simulink model "lim_s_function"  (R2017a)
settings: Solver=ode4  StartTime=0.0  StopTime=1  FixedStep=1e-5  MaxStep=1  RelTol=1e-3
settings Model: Creator=QAQ  LastModifiedBy=QAQ

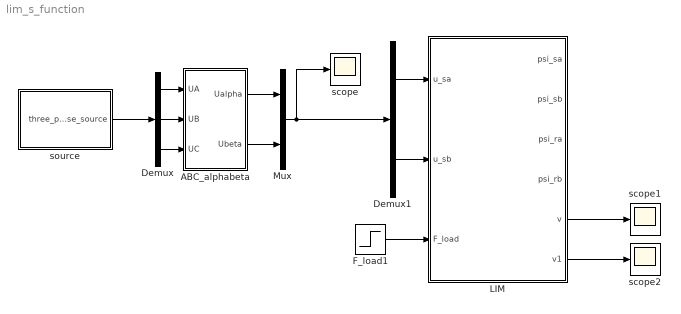
== system lim_s_function ==
  ABC_alphabeta : Subsystem
  Demux : Demux  Outputs=3
  Demux1 : Demux  Outputs=2
  F_load1 : Step  Time=0  After=1000  SampleTime=0
  LIM : Subsystem
  Mux : Mux  Inputs=2
  scope : Scope
  scope1 : Scope
  scope2 : Scope
  source : Subsystem
  wires:
  Demux/2 -> ABC_alphabeta/2(UB)
  Demux/3 -> ABC_alphabeta/3(UC)
  source/1(three_phase_source) -> Demux/1
  Mux/1 -> scope/1, Demux1/1
  ABC_alphabeta/2(Ubeta) -> Mux/2
  Demux/1 -> ABC_alphabeta/1(UA)
  Demux1/1 -> LIM/1(u_sa)
  ABC_alphabeta/1(Ualpha) -> Mux/1
  Demux1/2 -> LIM/2(u_sb)
  F_load1/1 -> LIM/3(F_load)
  LIM/5(v) -> scope1/1
  LIM/6(v1) -> scope2/1

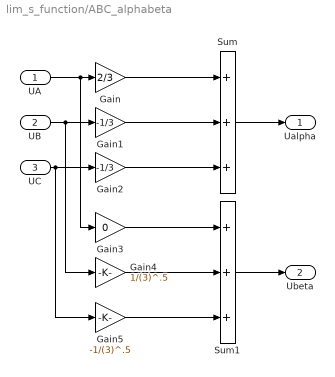
== system lim_s_function/ABC_alphabeta ==
  UA : Inport
  UB : Inport  Port=2
  UC : Inport  Port=3
  Gain : Gain  Gain=2/3  SaturateOnIntegerOverflow=on  OutDataTypeStr=Inherit: Same as input  ParamDataTypeStr=Inherit: Same as input
  Gain1 : Gain  Gain=-1/3  SaturateOnIntegerOverflow=on  OutDataTypeStr=Inherit: Same as input  ParamDataTypeStr=Inherit: Same as input
  Gain2 : Gain  Gain=-1/3  SaturateOnIntegerOverflow=on  OutDataTypeStr=Inherit: Same as input  ParamDataTypeStr=Inherit: Same as input
  Gain3 : Gain  Gain=0  SaturateOnIntegerOverflow=on  OutDataTypeStr=Inherit: Same as input  ParamDataTypeStr=Inherit: Same as input
  Gain4 : Gain  Gain=1/(3)^.5  SaturateOnIntegerOverflow=on  OutDataTypeStr=Inherit: Same as input  ParamDataTypeStr=Inherit: Same as input
  Gain5 : Gain  Gain=-1/(3)^.5  SaturateOnIntegerOverflow=on  OutDataTypeStr=Inherit: Same as input  ParamDataTypeStr=Inherit: Same as input
  Sum : Sum  Inputs=+++  SaturateOnIntegerOverflow=on
  Sum1 : Sum  Inputs=+++  SaturateOnIntegerOverflow=on
  Ualpha : Outport
  Ubeta : Outport  Port=2
  wires:
  UA/1 -> Gain3/1, Gain/1
  UB/1 -> Gain4/1, Gain1/1
  UC/1 -> Gain5/1, Gain2/1
  Gain/1 -> Sum/1
  Gain1/1 -> Sum/2
  Gain2/1 -> Sum/3
  Sum/1 -> Ualpha/1
  Gain3/1 -> Sum1/1
  Gain4/1 -> Sum1/2
  Gain5/1 -> Sum1/3
  Sum1/1 -> Ubeta/1

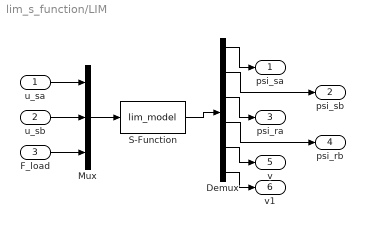
== system lim_s_function/LIM ==
  u_sa : Inport
  u_sb : Inport  Port=2
  F_load : Inport  Port=3
  Demux : Demux  Outputs=6
  Mux : Mux  Inputs=3
  S-Function : S-Function  FunctionName=lim_model  SFunctionDeploymentMode=off  EnableBusSupport=off
  psi_sa : Outport
  psi_sb : Outport  Port=2
  psi_ra : Outport  Port=3
  psi_rb : Outport  Port=4
  v : Outport  Port=5
  v1 : Outport  Port=6
  wires:
  Mux/1 -> S-Function/1
  u_sa/1 -> Mux/1
  u_sb/1 -> Mux/2
  F_load/1 -> Mux/3
  S-Function/1 -> Demux/1
  Demux/2 -> psi_sb/1
  Demux/1 -> psi_sa/1
  Demux/3 -> psi_ra/1
  Demux/5 -> v/1
  Demux/4 -> psi_rb/1
  Demux/6 -> v1/1

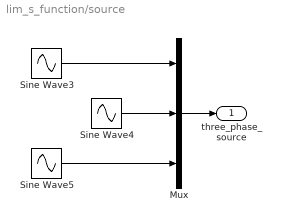
== system lim_s_function/source ==
  Mux : Mux  Inputs=3
  Sine Wave3 : Sin  Amplitude=500  Frequency=2*pi*50  SampleTime=0
  Sine Wave4 : Sin  Amplitude=500  Frequency=2*pi*50  Phase=-2*pi/3  SampleTime=0
  Sine Wave5 : Sin  Amplitude=500  Frequency=2*pi*50  Phase=2*pi/3  SampleTime=0
  three_phase_source : Outport
  wires:
  Sine Wave5/1 -> Mux/3
  Sine Wave3/1 -> Mux/1
  Mux/1 -> three_phase_source/1
  Sine Wave4/1 -> Mux/2
